simulink model "test_simulink2021"  (R2021a)
settings: Solver=VariableStepAuto  StartTime=0.0  StopTime=100  RelTol=1e-3
libraries: simulink_extras x1, vehdynlibsteering x1, autolibshared x1, simulink x1
settings Model: Creator=caugu  LastModifiedBy=caugu
settings DebuggingCC: UnconnectedInputMsg=none  UnconnectedOutputMsg=none  UnconnectedLineMsg=none
settings ModelReferenceCC: EnableRefExpFcnMdlSchedulingChecks=off
settings RTWCC: Description=Generic Real-Time Target  GPUComputeCapability=5.0  DLArmComputeVersion=20.02.1

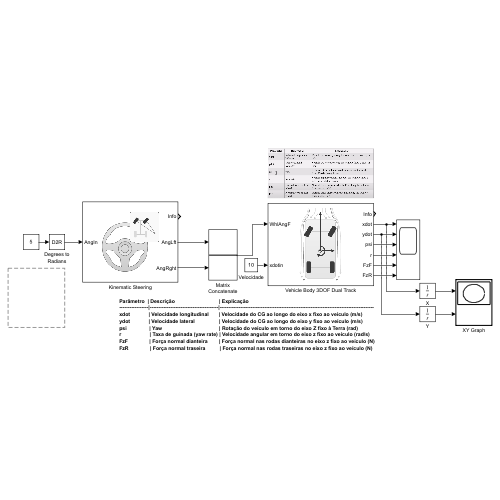
[thumbnail: Simulink's stored preview of the top-level diagram]
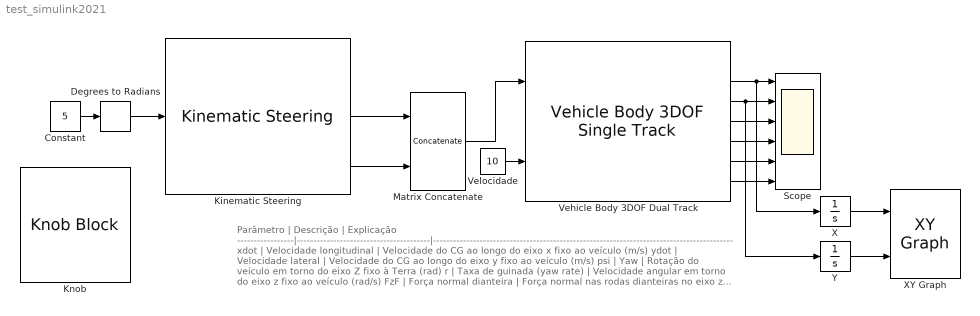
== system test_simulink2021 ==
  note: Parâmetro | Descrição | Explicação
      | -----------------|----------------------------------------|------------------------------------------------------------------------------------------
      | xdot | Velocidade longitudinal | Velocidade do CG ao longo do eixo x fixo ao veículo (m/s)
      | ydot | Velocidade lateral | Velocidade do CG ao longo do eixo y fixo ao veículo (m/s)
      | psi | Yaw | Rotação do veículo em torno do eixo Z fixo à Terra (rad)
      | r | Taxa de guinada (yaw rate) | Velocidade angular em torno do eixo z fixo ao veículo (rad/s)
      | FzF | Força normal dianteira | Força normal nas rodas dianteiras no eixo z fixo ao veículo (N)
      | FzR | Força normal traseira | Força normal nas rodas traseiras no eixo z fixo ao veículo (N)
  Constant : Constant  Value=5
  Degrees to Radians : simulink_extras/Transformations/Degrees to Radians
  Kinematic Steering : vehdynlibsteering/Kinematic Steering  StrgType=Ackerman  StrgRatioType=Constant  Loc=Front  NrmlFctr=0.01  TrckWdth=1  WhlBase=1.524  Db=0  StrgRng=1.25*pi  StrgAngBpts="[-6.2832   -5.0265   -3.7699   -2.5133   -1.2566         0    1.2566    2.5133    3.7699    5.0265    6.2832]"  StrgRatioTbl=|  StrgRatio=100  PctAckIn=off  PctAck=100  PctAckTbl=ones(1,11)*100  StrgArmLngth=0.1  RckCsLngth=0.5  TieRodLngth=0.248  D=0.2  PnnRadius=0.00085818  PnnRadiusTbl="[0.0055    0.0055    0.0056    0.0057    0.0058    0.0057    0.0057    0.0057    0.0056    0.0055    0.0055]"  RodLngth=0.1  ParaArmLngth=0.9  aMode=2
      | [13.5000   13.3750   13.2500   13.1250   13.0000   13.0000   13.0000   13.1250   13.2500   13.3750   13.5000
      | ]
  Knob : KnobBlock
  Matrix Concatenate : Concatenate  ConcatenateDimension=2
  Scope : Scope  NumInputPorts=6
  Vehicle Body 3DOF Dual Track : autolibshared/Vehicle Body 3DOF Single Track  trackMode=Dual  inputMode=External longitudinal velocity  frontSteerMode=on  rearSteerMode=off  windMode=off  muMode=off  extFMode=off  extMMode=off  htchFMode=off  htchMMode=off  extXo=off  extpsio=off  extxdoto=off  extro=off  extYo=off  extTamb=off  extydoto=off  aMode=2  NF=2  NR=2  m=2000  a=1.4  b=1.6  h=0.35  dh=1  hh=0.2  X_o=0  xdot_o=0  CalphaMode=off  sigmaMode=on  d=0  hl=0  w=[1.4,1.4]  Cy_f=12e3  Cy_r=11e3  sigma_f=.1  sigma_r=.1  alpha_f_brk=[-.1 .1]  Cy_f_data=[-9e3 9e3]  alpha_r_brk=[-.1 .1]  Cy_r_data=[-9e3 9e3]  Y_o=0  ydot_o=0  Izz=4000  psi_o=0  r_o=0  Af=2  Cd=.3  Cl=.1  Cpm=.1  beta_w=[0 0.01:0.01:0.3]  Cs=[0:0.03:0.9]  Cym=[0 1e-6:0.01:0.3]  Pabs=101325  Tair=273  g=9.81  mu=1  xdot_tol=.01  Fznom=5000  Fxtire_sat=7e4  Fytire_sat=7e4  longOff=0  latOff=0  vertOff=0  wrapAng=off
  Velocidade : Constant  Value=10
  X : Integrator
  XY Graph : simulink/Sinks/XY Graph  xmin=-1  xmax=1  ymin=-1  ymax=1  st=-1
  Y : Integrator
  wires:
  Degrees to Radians/1 -> Kinematic Steering/1
  Kinematic Steering/2 -> Matrix Concatenate/1
  Kinematic Steering/3 -> Matrix Concatenate/2
  Matrix Concatenate/1 -> Vehicle Body 3DOF Dual Track/1
  Vehicle Body 3DOF Dual Track/2 -> X/1, Scope/1
  Vehicle Body 3DOF Dual Track/3 -> Y/1, Scope/2
  Vehicle Body 3DOF Dual Track/4 -> Scope/3
  Vehicle Body 3DOF Dual Track/5 -> Scope/4
  Vehicle Body 3DOF Dual Track/6 -> Scope/5
  Vehicle Body 3DOF Dual Track/7 -> Scope/6
  Constant/1 -> Degrees to Radians/1
  Velocidade/1 -> Vehicle Body 3DOF Dual Track/2
  X/1 -> XY Graph/1
  Y/1 -> XY Graph/2
